simulink model "cartesian_control_loop"  (R2014a)
settings: Solver=ode45  StartTime=0.0  StopTime=10  MaxStep=0.001  RelTol=1e-3
values from neighbouring files (symbols this model uses):
  sin_omega = sin_freq * 2 * pi    (= 0.314159265359)    [cartesian_control_parameters.m]
  v_max = 0.25e3    (= 250)    [cartesian_control_parameters.m]
settings Model: Creator=yezhongyi  LastModifiedBy=andy
settings DataIOCC: SignalLoggingSaveFormat=ModelDataLogs
settings DebuggingCC: MultiTaskDSMMsg=warning  MultiTaskCondExecSysMsg=none
settings RTWCC: IncludeERTFirstTime=on

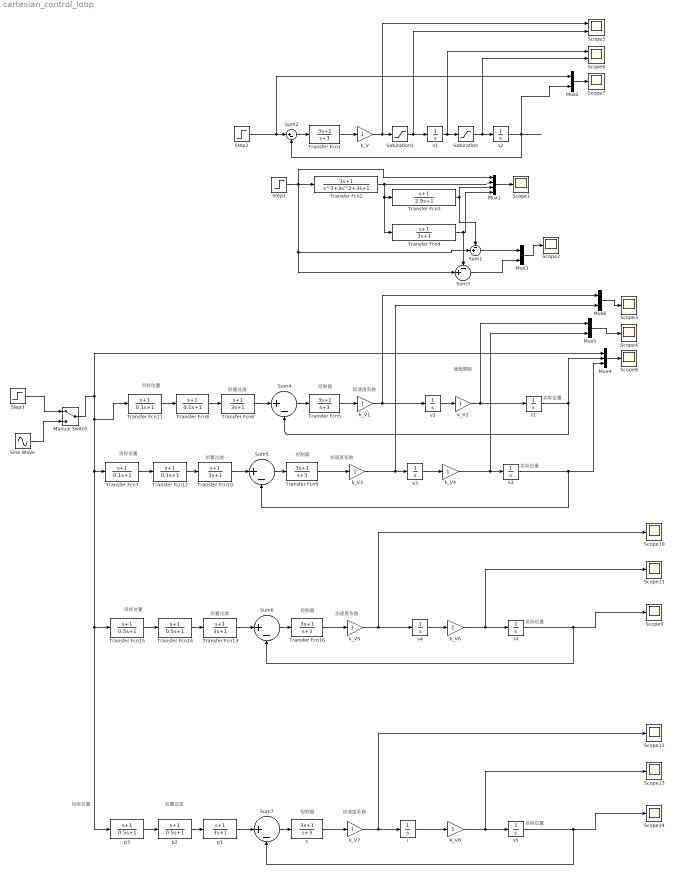
== system cartesian_control_loop ==
  note: 加速度系数
  note: 控制器
  note: 速度限制
  note: 前置过滤
  note: 目标位置
  note: 实际位置
  note: 加速度系数
  note: 控制器
  note: 前置过滤
  note: 目标位置
  note: 实际位置
  note: 加速度系数
  note: 控制器
  note: 前置过滤
  note: 目标位置
  note: 实际位置
  note: 加速度系数
  note: 控制器
  note: 前置过滤
  note: 目标位置
  note: 实际位置
  Manual Switch : ManualSwitch
  Mux1 : Mux
  Mux{2..3,5..6} (4 alike) : Mux  Inputs=2
  Mux4 : Mux  Inputs=3
  Saturation : Saturate  UpperLimit=0.4  LowerLimit=-0.4
  Saturation1 : Saturate  UpperLimit=0.4  LowerLimit=-0.4
  Scope{1..4,7..14} (12 alike) : Scope
      Scope10 settings: SaveName=ScopeData9
      Scope11 settings: SaveName=ScopeData10
      Scope12 settings: SaveName=ScopeData11
      Scope13 settings: SaveName=ScopeData12
      Scope14 settings: SaveName=ScopeData13
      Scope3 settings: SaveName=ScopeData2
      Scope4 settings: SaveName=ScopeData3
      Scope7 settings: SaveName=ScopeData7
      Scope8 settings: SaveName=ScopeData4
      Scope9 settings: SaveName=ScopeData8
  Scope5 : Scope  NumInputPorts=2
      settings: YMin=-5~-5  YMax=5~5  SaveName=ScopeData5
  Scope6 : Scope  NumInputPorts=2
      settings: YMin=-5~-5  YMax=5~5  SaveName=ScopeData6
  Sine Wave : Sin  Frequency=sin_omega  SampleTime=0
  Step1 : Step  Time=0.001  After=0.4  SampleTime=0
  Step2 : Step  Time=0.001  After=0.4  SampleTime=0
  Step3 : Step  Time=0.001  After=400  SampleTime=0
  Sum1 : Sum  Inputs=-+|
  Sum{2,4..7} (5 alike) : Sum  Inputs=|+-
  Sum3 : Sum  Inputs=-+|
  Transfer Fcn{1,5,9,16} (4 alike) : TransferFcn  Numerator=[3 1]  Denominator=[1 3]
  Transfer Fcn10 : TransferFcn  Numerator=[1, 1]  Denominator=[3 1]
  Transfer Fcn{7..8,11..12} (4 alike) : TransferFcn  Numerator=[1, 1]  Denominator=[0.1 1]
  Transfer Fcn13 : TransferFcn  Numerator=[1, 1]  Denominator=[3 1]
  Transfer Fcn14 : TransferFcn  Numerator=[1, 1]  Denominator=[0.5 1]
  Transfer Fcn15 : TransferFcn  Numerator=[1, 1]  Denominator=[0.5 1]
  Transfer Fcn2 : TransferFcn  Numerator=[3 1]  Denominator=[1 3 3 1]
  Transfer Fcn3 : TransferFcn  Numerator=[1 1]  Denominator=[2.9 1]
  Transfer Fcn4 : TransferFcn  Numerator=[1 1]  Denominator=[3 1]
  Transfer Fcn6 : TransferFcn  Numerator=[1, 1]  Denominator=[3 1]
  c : TransferFcn  Numerator=[3 1]  Denominator=[1 3]
  i : Integrator  LimitOutput=on  UpperSaturationLimit=v_max  LowerSaturationLimit=-v_max
  k_V{,1..8} (9 alike) : Gain
  p1 : TransferFcn  Numerator=[1, 1]  Denominator=[3 1]
  p2 : TransferFcn  Numerator=[1, 1]  Denominator=[0.5 1]
  p3 : TransferFcn  Numerator=[1, 1]  Denominator=[0.5 1]
  s{1..5} (5 alike) : Integrator
  v1 : Integrator
  v2 : Integrator  LimitOutput=on  UpperSaturationLimit=v_max  LowerSaturationLimit=-v_max
  v3 : Integrator  UpperSaturationLimit=v_max  LowerSaturationLimit=-v_max
  v4 : Integrator  LimitOutput=on  UpperSaturationLimit=v_max  LowerSaturationLimit=-v_max
  wires:
  Transfer Fcn1/1 -> k_V/1
  k_V/1 -> Saturation1/1, Scope5/1
  v1/1 -> Saturation/1, Scope6/1
  s2/1 -> Mux2/2, Sum2/2
  Sum2/1 -> Transfer Fcn1/1
  Step2/1 -> Mux2/1, Sum2/1
  Mux2/1 -> Scope7/1
  Step1/1 -> Sum3/2, Sum1/2, Mux1/1, Transfer Fcn2/1
  Transfer Fcn2/1 -> Transfer Fcn4/1, Transfer Fcn3/1, Mux1/2
  Mux1/1 -> Scope1/1
  Transfer Fcn3/1 -> Sum1/1, Mux1/3
  Sum1/1 -> Mux3/1
  Transfer Fcn4/1 -> Mux1/4, Sum3/1
  Mux3/1 -> Scope2/1
  Sum3/1 -> Mux3/2
  Saturation/1 -> Scope6/2, s2/1
  Saturation1/1 -> Scope5/2, v1/1
  Transfer Fcn5/1 -> k_V1/1
  s1/1 -> Sum4/2, Mux4/2
  Sum4/1 -> Transfer Fcn5/1
  Mux4/1 -> Scope8/1
  k_V2/1 -> s1/1, Mux5/1
  Transfer Fcn6/1 -> Sum4/1
  Mux5/1 -> Scope4/1
  Mux6/1 -> Scope3/1
  k_V1/1 -> v2/1, Mux6/1
  v2/1 -> k_V2/1
  Transfer Fcn8/1 -> Transfer Fcn6/1
  Transfer Fcn11/1 -> Transfer Fcn8/1
  Step3/1 -> Manual Switch/1
  Sine Wave/1 -> Manual Switch/2
  Transfer Fcn9/1 -> k_V3/1
  s3/1 -> Mux4/3, Sum5/2
  Sum5/1 -> Transfer Fcn9/1
  k_V4/1 -> Mux5/2, s3/1
  Transfer Fcn10/1 -> Sum5/1
  k_V3/1 -> Mux6/2, v3/1
  v3/1 -> k_V4/1
  Transfer Fcn12/1 -> Transfer Fcn10/1
  Transfer Fcn7/1 -> Transfer Fcn12/1
  Transfer Fcn16/1 -> k_V5/1
  s4/1 -> Scope9/1, Sum6/2
  Sum6/1 -> Transfer Fcn16/1
  k_V6/1 -> Scope11/1, s4/1
  Transfer Fcn13/1 -> Sum6/1
  k_V5/1 -> Scope10/1, v4/1
  v4/1 -> k_V6/1
  Transfer Fcn14/1 -> Transfer Fcn13/1
  Transfer Fcn15/1 -> Transfer Fcn14/1
  c/1 -> k_V7/1
  s5/1 -> Scope14/1, Sum7/2
  Sum7/1 -> c/1
  k_V8/1 -> Scope13/1, s5/1
  p1/1 -> Sum7/1
  k_V7/1 -> Scope12/1, i/1
  i/1 -> k_V8/1
  Manual Switch/1 -> p3/1, Transfer Fcn15/1, Transfer Fcn7/1, Transfer Fcn11/1, Mux4/1
  p2/1 -> p1/1
  p3/1 -> p2/1
